simulink model "m1_B_Sumulink"  (R2022b)
settings: Solver=ode45  StartTime=0.0  StopTime=10.0  MaxStep=0.01  RelTol=1e-3
settings Model: Creator=Asus  LastModifiedBy=ThinkPad

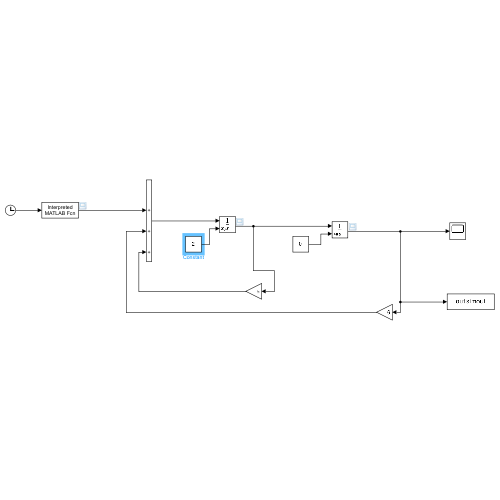
[thumbnail: Simulink's stored preview of the top-level diagram]
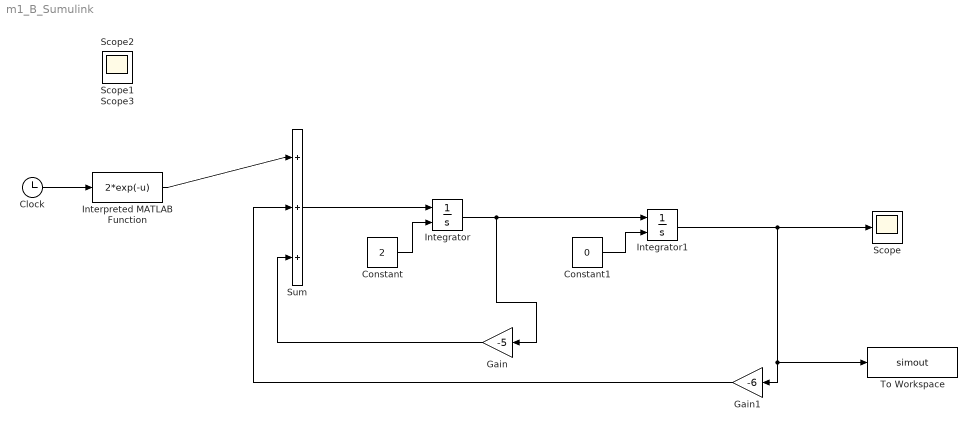
== system m1_B_Sumulink ==
  Clock : Clock
  Constant : Constant  Value=2
  Constant1 : Constant  Value=0
  Gain : Gain  Gain=-5
  Gain1 : Gain  Gain=-6
  Integrator : Integrator  InitialConditionSource=external
  Integrator1 : Integrator  InitialConditionSource=external
  Interpreted MATLAB Function : MATLABFcn  MATLABFcn=2*exp(-u)
  Scope{,1..3} (4 alike) : Scope
  Sum : Sum  Inputs=|+++
  To Workspace : ToWorkspace  VariableName=simout  SaveFormat=Timeseries  SampleTime=-1
  wires:
  Constant/1 -> Integrator/2
  Sum/1 -> Integrator/1
  Constant1/1 -> Integrator1/2
  Integrator/1 -> Gain/1, Integrator1/1
  Gain/1 -> Sum/3
  Integrator1/1 -> Scope/1, To Workspace/1, Gain1/1
  Gain1/1 -> Sum/2
  Clock/1 -> Interpreted MATLAB Function/1
  Interpreted MATLAB Function/1 -> Sum/1
